simulink model "LimitedSlipDifferentialWithClutches"  (R2023a)
settings: Solver=VariableStepAuto  StartTime=0.0  StopTime=Sim_Time  FixedStep=1e-3  RelTol=1e-3  AbsTol=1e-3  EnableMultiTasking=on
model workspace (MATLAB code in the model file):
  | MFormulaCoeff.DryTarmac = [10 1.9 1 0.97];
  | MFormulaCoeff.WetTarmac = [12 2.3 0.82 1];
  | MFormulaCoeff.Snow         = [5 2 0.3 1];
  | MFormulaCoeff.Ice            = [4 2 0.1 1];
libraries: fl_lib x46, nesl_utility x14, sdl_lib x11, simulink x1
(part 1 of 2)
CloseFcn:
  | try,close(h1_LimitedSlipDifferentialWithClutches),end
  | clear h1_LimitedSlipDifferentialWithClutches
  | try,close(h2_LimitedSlipDifferentialWithClutches),end
  | clear h2_LimitedSlipDifferentialWithClutches
  | 
  | clear simlog_LimitedSlipDifferentialWithClutches
  | clear logsout_LimitedSlipDifferentialWithClutches
Description:
  | Limited Slip Differential with Clutches
settings Model: Creator=The MathWorks, Inc.  LastModifiedBy=MCO
settings SolverCC: AutoScaleAbsTol=off  ZcThreshold=0  MaxConsecutiveZCs=100  MaxConsecutiveMinStep=10  ZeroCrossAlgorithm=Adaptive  AlgebraicLoopSolver=TrustRegion
settings DataIOCC: LimitDataPoints=on  MaxDataPoints=10000  SaveOutput=off  DSMLogging=off  ReturnWorkspaceOutputs=off  SignalLoggingName=logsout_LimitedSlipDifferentialWithClutches
settings OptimizationCC: ExpressionDepthLimit=2147483647  InitFltsAndDblsToZero=on  EfficientMapNaN2IntZero=off  LifeSpan=inf
settings DebuggingCC: SaveWithDisabledLinksMsg=none  SaveWithParameterizedLinksMsg=none  SignalResolutionControl=TryResolveAllWithWarning  MaxConsecutiveZCsMsg=none  IgnoredZcDiagnostic=none  UnconnectedInputMsg=warning  UnconnectedOutputMsg=warning  UnconnectedLineMsg=warning  StateNameClashWarn=warning  SFUnexpectedBacktrackingDiag=warning  SFNoUnconditionalDefaultTransitionDiag=warning  SFExecutionAtInitializationDiag=none  ArithmeticOperatorsInVariantConditions=warning
settings HardwareCC: ProdBitPerPointer=32  ProdBitPerSizeT=32  ProdBitPerPtrDiffT=32  ProdLargestAtomicFloat=None  ProdIntDivRoundTo=Undefined  ProdEndianess=Unspecified  ProdWordSize=32  ProdHWDeviceType=32-bit Generic
settings ModelReferenceCC: EnableRefExpFcnMdlSchedulingChecks=on  PropagateSignalLabelsOutOfModel=off
settings SFSimCC: SimUseLocalCustomCode=off  CustomCodeUndefinedFunction=UseInterfaceOnly
settings RTWCC: RTWUseLocalCustomCode=off  DLArmComputeVersion=19.05
settings CodeAppCC: StateflowObjectComments=on
settings GRTTargetCC: TargetFcnLib=ansi_tfl_tmw.mat  TargetLangStandard=C89/C90 (ANSI)  CombineOutputUpdateFcns=off  GRTInterface=on
settings ConfigComp: CovMetricSettings=dw  CovSaveCumulativeToWorkspaceVar=on  CovSaveSingleToWorkspaceVar=on  CovExternalEMLEnable=off
settings SimscapeCC: SimscapeLogType=all  SimscapeLogSimulationStatistics=on  SimscapeLogName=simlog_LimitedSlipDifferentialWithClutches  SimscapeLogDataHistory=10000

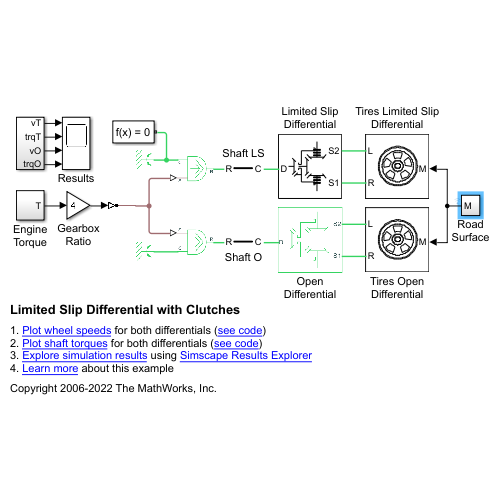
[thumbnail: Simulink's stored preview of the top-level diagram]
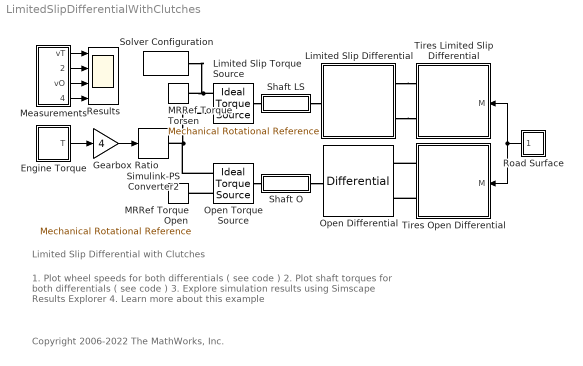
== system LimitedSlipDifferentialWithClutches ==
  note: Limited Slip Differential with Clutches
  note: 1. Plot wheel speeds for both differentials ( see code )
      | 2. Plot shaft torques for both differentials ( see code )
      | 3. Explore simulation results using Simscape Results Explorer
      | 4. Learn more about this example
  note: Copyright 2006-2022 The MathWorks, Inc.
  Engine Torque : Subsystem
  Gearbox Ratio : Gain  Gain=4  SaturateOnIntegerOverflow=on  OutDataTypeStr=Inherit: Same as input  ParamDataTypeStr=Inherit: Same as input
  Limited Slip Differential : Subsystem  Tag=PublishSubsystem
      mask Display:
      | plot([73.6983027309179;73.6983027309179], [209.756707772613;130.389304831624])
      | plot([73.6983027309179;39.6837014704943], [170.073006302118;170.073006302118])
      | plot([62.3601023107767;85.0365031510592], [221.094908192754;198.418507352471])
      | plot([85.0365031510592;62.3601023107767], [141.727505251765;119.051104411483])
      | plot([102.043803781271;119.051104411483;119.051104411483;198.418507352471;198.418507352471], [181.41120672226;181.41120672226;260.778609663248;260.778609663248;277.78591029346])
      | patch([80 120 120 80 80]+115,[150 150 155 155 150]+80,[0 0 0]);
      | patch([80 120 120 80 80]+115,[150 150 155 155 150]+95,[0 0 0]);
      | patch([80 120 120 80 80]+115,[150 150 155 155 150]+110,[0 0 0]);
      | patch([80 120 120 80 80]+115,[150 150 155 155 150]-80,[0 0 0]);
      | patch([80 120 120 80 80]+115,[150 150 155 155 150]-65,[0 0 0]);
      | patch([80 120 120 80 80]+115,[150 150 155 155 150]-50,[0 0 0]);
      | 
      | plot([164.403906092048;255.109509453177], [226.764008402824;226.764008402824])
      | plot([153.065705671906;153.065705671906], [215.425807982683;124.720204621553])
      | plot([209.756707772613;209.756707772613], [317.469611763954;226.764008402824])
      | plot([187.08030693233;198.418507352471], [277.78591029346;277.78591029346])
      | plot([141.727505251765;164.403906092048], [226.764008402824;204.087607562542])
      | plot([175.742106512189;153.065705671906], [124.720204621553;102.043803781271])
      | plot([153.065705671906;175.742106512189], [238.102208822966;215.425807982683])
      | plot([209.756707772613;209.756707772613], [113.382004201412;22.6764008402824])
      | plot([164.403906092048;141.727505251765], [136.058405041695;113.382004201412])
      | plot([243.771309033036;266.447709873319], [124.720204621553;102.043803781271])
      | plot([266.447709873319;243.771309033036], [238.102208822966;215.425807982683])
      | plot([164.403906092048;255.109509453177], [113.382004201412;113.382004201412])
      | plot([187.08030693233;198.418507352471;198.418507352471;119.051104411483;119.051104411483;102.043803781271;102.043803781271], [62.3601023107767;62.3601023107767;79.3674029409885;79.3674029409885;158.734805881977;158.734805881977;147.396605461836])
      | plot([102.043803781271;153.065705671906], [170.073006302118;170.073006302118])
      | plot([102.043803781271;102.043803781271], [181.41120672226;192.749407142401])
      | plot([96.3747035712004;73.6983027309179], [130.389304831624;107.712903991342])
      | plot([85.0365031510592;119.051104411483], [119.051104411483;119.051104411483])
      | plot([-20;-20;360.146012604237;360.146012604237;-20], [360.146012604237;-20;-20;360.146012604237;360.146012604237])
  Limited Slip Torque Source : fl_lib/Mechanical/Mechanical Sources/Ideal Torque Source
  MRRef Torque Open : fl_lib/Mechanical/Rotational Elements/Mechanical Rotational Reference
  MRRef Torque Torsen : fl_lib/Mechanical/Rotational Elements/Mechanical Rotational Reference
  Measurements : Subsystem
  Open Differential : sdl_lib/Gears/Differential  driveshaft_location=2  cd_ratio=1.33  friction_model=1  efficiency=[ 0.9 0.92 ]  temperature_TLU=[ 280 300 320 ] K  efficiency_ss_TLU=[ 0.95 0.9 0.85 ]  efficiency_cd_TLU=[ 0.95 0.9 0.85 ]  pwr_thr=[ 0.001 0.001 ] W  mu_visc=[ 0 0 ] N*m/(rad/s)  model_inertia=0  carrier_inertia=0.001 kg*m^2  planet_inertia=0.001 kg*m^2  thermal_mass=50 J/K  T_init=300 K
  Open Torque Source : fl_lib/Mechanical/Mechanical Sources/Ideal Torque Source
  Results : Scope  NumInputPorts=4
  Road Surface : Subsystem
  Shaft LS : Subsystem
      mask Display:
      | patch([-1 -1 1 1 -1]*25,[-1 1 1 -1 -1]*5,[1 1 1]);
      | patch([-1 -1 1 1 -1]*11,[-1 1 1 -1 -1]*0.1,[0 0 0]);
  Shaft O : Subsystem
      mask Display:
      | patch([-1 -1 1 1 -1]*25,[-1 1 1 -1 -1]*5,[1 1 1]);
      | patch([-1 -1 1 1 -1]*11,[-1 1 1 -1 -1]*0.1,[0 0 0]);
  Simulink-PS Converter2 : nesl_utility/Simulink-PS Converter  PhysicalDomain=network_engine_domain  SubClassName=ps_input  LeftPortType=input  RightPortType=output  PseudoPeriodic=off  Frequencies=[]  NoiseDistribution=none  NoiseParameters=[]  Unit=1  AffineConversion=off  FilteringAndDerivatives=filter  SimscapeFilterOrder=1  InputFilterTimeConstant=0.001  UdotUserProvided=0
  Solver Configuration : nesl_utility/Solver Configuration  PhysicalDomain=network_engine_domain  SubClassName=solver  LeftPortType=input  RightPortType=generic  Tones=[]  Harmonics=[]  SimulateNoise=off  Profile=off  UseLocalSampling=off  EnableSwitchedLinearOptims=on  FrequencyDomain=off  UseCCode=off  RelTol=0.001  AbsTol=1e-06  MinStep=1e-09  ToWorkspace=off  RevertToSquareIcSolve=off  NumHomotopyIterations=100  PhasorMode=off  PhasorModeNumHarmonics=1  ConsistencySolver=NEWTON_XTOL_AFTER_FTOL  IndexReductionMethod=DerivativeReplacement  DoDC=off  ResidualTolerance=1e-9  ConsistencyTolSource=GLOBAL  ConsistencyAbsTol=0.001  ConsistencyRelTol=0.001  ConsistencyTolFactor=0.001  UseLocalSolver=off  LocalSolverChoice=NE_BACKWARD_EULER_ADVANCER  ResolveIndetEquations=on  FunctionEvalNumThread=1  LocalSolverSampleTime=.001  DoFixedCost=off  MaxNonlinIter=12  MaxModeIter=2  ComputeImpulses=off  ImpulseIterations=2  LinearAlgebra=auto  LinearAlgebraNumThread=0  EquationFormulation=NE_TIME_EF  DelaysMemoryBudget=1024  AutomaticFiltering=on  FilteringTimeConstant=0.001  PartitionStorageMethod=AS_NEEDED  PartitionMemoryBudget=1024  PartitionMethod=FAST
  Tires Limited Slip Differential : Subsystem  Tag=PublishSubsystem
      mask Display:
      | plot([199.740630080105;207.645625381422;215.666495494822;223.725995056458;231.746506679781;239.614636200368], [285.533592122614;287.104128914395;287.892278108498;287.890449397339;287.098660392404;285.533592122614])
      | plot([182.29422131887;191.284049604609;200.547323621308;209.994832976365;219.535592990157;229.077720928241;238.529320882316;247.799368778054;256.798588986696;257.061044961602], [327.86290499758;331.09432156677;333.429020721321;334.844518032099;335.327181486212;334.872362770745;333.484442038558;331.176785725016;327.971617821912;327.86290499758])
      | plot([182.293066754937;199.741297401488], [327.862962149084;285.533680580556])
      | plot([239.613968878984;257.062199525535], [285.533680580556;327.862962149084])
      | plot([161.12998329239;162.078783791624;163.80431860203;166.28996988011;169.511799445263;173.438779317544;173.475674844307], [230.482414304504;238.453500201144;246.293204428793;253.926026350122;261.278457717503;268.279690597622;268.338450605791])
      | plot([115.521208412501;115.19363189143;115.795069625231;117.319729439748;119.752928027503;123.071232355974;127.242685340509;132.227113608518;137.976514391014;138.639091794056], [226.950718692202;236.412705455625;245.861238280392;255.205322630308;264.354969865087;273.222063880151;281.72120971289;289.770555942828;297.29258296555;298.068153121848])
      | plot([115.523664280772;161.128425970674], [226.952978409827;230.480418540537])
      | plot([173.474466428161;138.640995137393], [268.337409943342;298.068691045046])
      | plot([197.791294323752;190.505905487348;183.583957764389;177.092113295368;171.092892091325;165.644069931963;165.540704869119], [173.730032993176;177.080059057945;181.128046811489;185.835011918887;191.155623733067;197.038641853715;197.162104079289])
      | plot([187.018154556423;177.935574592276;169.151745387891;160.751260020237;152.815019755577;145.419454926048;138.635788863788;132.529351981303;127.158952603892;126.547993304079], [129.256249226993;131.857994736568;135.337460645285;139.661137794374;144.787386809327;150.666839109836;157.242872356214;164.45215575347;172.225259961496;173.223046112601])
      | plot([187.017316929996;197.78860732913], [129.25548478961;173.726426437497])
      | plot([165.537726134062;126.546914689243], [197.158707305789;173.222506418824])
      | plot([269.470357644972;273.38551933114;276.602305486856;279.089736702965;280.82385765709;281.787967816474;281.81616724833], [262.922159053497;255.989463868491;248.706398553292;241.143103008215;233.372415903877;225.469173204983;225.06588742066])
      | plot([304.431346528147;310.265227080294;315.332070863713;319.583081402952;322.977319142679;325.482095717982;327.073288761189;327.735574213461;327.462573903851;327.423015855416], [292.655530476138;285.116593543042;277.042138363134;268.509926353743;259.602127380701;250.404528417616;241.005707370423;231.496180023723;221.967528324303;221.475771485887])
      | plot([304.430681280792;269.471229985356], [292.651550844312;262.920269742608])
      | plot([281.817270442843;327.422032132745], [225.063278339803;221.472848206758])
      | plot([274.506490288884;269.03580586378;263.012187571475;256.493646148968;249.542958713556;242.227064184873;242.193171590222], [197.094155985096;191.184202827407;185.838928552521;181.109811073729;177.042394377551;173.675849910247;173.662235378073])
      | plot([313.374602600377;308.147922202874;302.181086731703;295.531560074253;288.263380807238;280.446545470191;272.156334460522;263.472587042146;254.478932449722;252.966160341391], [173.157457637183;165.349405231175;158.09125499764;151.452906891035;145.498291832517;140.284756020223;135.862508654033;132.274138393531;129.554203205929;129.189658564058])
      | plot([313.375261612236;274.510430172086], [173.15951641649;197.095717303455])
      | plot([242.196558974683;252.967849373817], [173.663436435163;129.192494787276])
      | plot([371.389053761959;370.658673461755;368.474566522701;364.857767088574;359.843106915069;353.478879920948;345.826377091206;336.959296211375;326.963032117569;315.933854297525;303.977979762811;291.210550120943;277.754522698759;263.739486396147;249.3004136741;234.576360696131;219.709128141403;204.841895586676;190.117842608706;175.678769886659;161.663733584047;148.207706161863;135.440276519995;123.484401985281;112.455224165237;102.458960071431;93.5918791916006;85.939376361858;79.5751493677372;74.5604891942319;70.9436897601051;68.7595828210511;68.0292025208473;68.7595828210511;70.9436897601053;74.5604891942321;79.5751493677375;85.9393763618583;93.5918791916009;102.458960071431;112.455224165237;123.484401985282;135.440276519995;148.207706161863;161.663733584048;175.67876988666;190.117842608707;204.841895586676;219.709128141403;234.576360696131;249.3004136741;263.739486396147;277.754522698759;291.210550120943;303.977979762811;315.933854297525;326.963032117569;336.959296211375;345.826377091205;353.478879920948;359.843106915069;364.857767088574;368.474566522701;370.658673461755;371.389053761959;371.389053761959;371.389053761959], [228.149788454175;213.282555899448;198.558502921478;184.119430199431;170.104393896819;156.648366474635;143.880936832767;131.925062298053;120.895884478009;110.899620384203;102.032539504372;94.3800366746299;88.0158096805091;83.0011495070038;79.3843500728769;77.2002431338229;76.4698628336191;77.2002431338229;79.3843500728769;83.0011495070038;88.0158096805092;94.38003667463;102.032539504373;110.899620384203;120.895884478009;131.925062298053;143.880936832767;156.648366474635;170.104393896819;184.119430199431;198.558502921479;213.282555899448;228.149788454175;243.017021008903;257.741073986872;272.180146708919;286.195183011531;299.651210433715;312.418640075584;324.374514610297;335.403692430341;345.399956524147;354.267037403978;361.91954023372;368.283767227841;373.298427401346;376.915226835473;379.099333774527;379.829714074731;379.099333774527;376.915226835473;373.298427401346;368.283767227841;361.91954023372;354.267037403978;345.399956524147;335.403692430341;324.374514610297;312.418640075583;299.651210433715;286.195183011531;272.180146708919;257.741073986872;243.017021008903;228.149788454176;228.149788454175;228.149788454175])
      | plot([363.45231346786;362.760150741504;360.690328467866;357.26278016692;352.510515002494;346.479299885972;339.227218715925;330.824112998412;321.350909235096;310.898839556798;299.568563108203;287.46919664527;274.717263681223;261.435572301422;247.752032454366;233.798424108965;219.709128141403;205.619832173842;191.666223828441;177.982683981384;164.700992601583;151.949059637537;139.849693174603;128.519416726008;118.067347047711;108.594143284395;100.191037566881;92.9389563968342;86.9077412803127;82.1554761158862;78.7279278149405;76.6581055413021;75.9659428149462;76.6581055413021;78.7279278149406;82.1554761158864;86.907741280313;92.9389563968345;100.191037566881;108.594143284395;118.067347047711;128.519416726009;139.849693174604;151.949059637537;164.700992601584;177.982683981384;191.666223828441;205.619832173842;219.709128141403;233.798424108965;247.752032454366;261.435572301422;274.717263681223;287.46919664527;299.568563108203;310.898839556798;321.350909235095;330.824112998411;339.227218715925;346.479299885972;352.510515002493;357.26278016692;360.690328467866;362.760150741504;363.45231346786;363.45231346786;363.45231346786], [228.149788454175;214.060492486614;200.106884141213;186.423344294156;173.141652914355;160.389719950309;148.290353487375;136.96007703878;126.508007360483;117.034803597167;108.631697879653;101.379616709606;95.3484015930846;90.596136428658;87.1685881277123;85.0987658540739;84.406603127718;85.0987658540739;87.1685881277124;90.5961364286582;95.3484015930846;101.379616709606;108.631697879653;117.034803597167;126.508007360483;136.960077038781;148.290353487376;160.389719950309;173.141652914355;186.423344294156;200.106884141213;214.060492486614;228.149788454175;242.239084421737;256.192692767138;269.876232614194;283.157923993995;295.909856958042;308.009223420975;319.33949986957;329.791569547868;339.264773311184;347.667879028697;354.919960198744;360.951175315265;365.703440479692;369.130988780638;371.200811054276;371.892973780632;371.200811054276;369.130988780638;365.703440479692;360.951175315265;354.919960198744;347.667879028697;339.264773311184;329.791569547868;319.33949986957;308.009223420975;295.909856958042;283.157923993995;269.876232614194;256.192692767138;242.239084421737;228.149788454176;228.149788454175;228.149788454175])
      | plot([261.408509686589;261.209838965396;260.615740109466;259.631934615548;258.267897068353;256.536763895118;254.455206854636;252.043272479101;249.324189015046;246.324142722634;243.072025687652;239.599157574934;235.93898400287;232.126754443812;228.199182752392;224.194093591025;220.150058157742;216.106022724459;212.100933563092;208.173361871672;204.361132312614;200.70095874055;197.228090627832;193.97597359285;190.975927300438;188.256843836383;185.844909460848;183.763352420366;182.032219247131;180.668181699936;179.684376206018;179.090277350088;178.891606628895;179.090277350088;179.684376206019;180.668181699936;182.032219247131;183.763352420366;185.844909460848;188.256843836383;190.975927300438;193.97597359285;197.228090627833;200.70095874055;204.361132312614;208.173361871672;212.100933563092;216.106022724459;220.150058157742;224.194093591025;228.199182752392;232.126754443812;235.93898400287;239.599157574934;243.072025687652;246.324142722634;249.324189015046;252.043272479101;254.455206854636;256.536763895118;258.267897068353;259.631934615548;260.615740109465;261.209838965396;261.408509686589;261.408509686589], [229.220618493855;225.176583060572;221.171493899205;217.243922207785;213.431692648727;209.771519076663;206.298650963945;203.046533928963;200.046487636551;197.327404172496;194.915469796961;192.833912756479;191.102779583244;189.738742036049;188.754936542131;188.160837686201;187.962166965008;188.160837686201;188.754936542131;189.738742036049;191.102779583244;192.833912756479;194.915469796961;197.327404172496;200.046487636551;203.046533928963;206.298650963945;209.771519076663;213.431692648727;217.243922207785;221.171493899205;225.176583060572;229.220618493855;233.264653927138;237.269743088505;241.197314779925;245.009544338983;248.669717911047;252.142586023765;255.394703058747;258.394749351159;261.113832815214;263.525767190749;265.607324231231;267.338457404466;268.702494951661;269.686300445579;270.280399301509;270.479070022702;270.280399301509;269.686300445579;268.702494951661;267.338457404466;265.607324231231;263.525767190749;261.113832815214;258.394749351159;255.394703058747;252.142586023765;248.669717911047;245.009544338983;241.197314779925;237.269743088505;233.264653927139;229.220618493855;229.220618493855])
      | plot([240.243868902326;240.144988512846;239.849299616612;239.359649859334;238.680754835845;237.819152676342;236.783141080621;235.58269740669;234.229382583359;232.736229772174;231.117618850946;229.38913792767;227.56743321852;225.670048735692;223.715257328969;221.721884708198;219.709128141403;217.696371574609;215.702998953837;213.748207547115;211.850823064286;210.029118355137;208.30063743186;206.682026510633;205.188873699447;203.835558876116;202.635115202186;201.599103606465;200.737501446962;200.058606423472;199.568956666194;199.27326776996;199.174387380481;199.27326776996;199.568956666194;200.058606423472;200.737501446962;201.599103606465;202.635115202186;203.835558876116;205.188873699447;206.682026510633;208.30063743186;210.029118355137;211.850823064286;213.748207547115;215.702998953837;217.696371574609;219.709128141403;221.721884708198;223.715257328969;225.670048735692;227.56743321852;229.38913792767;231.117618850946;232.736229772174;234.229382583359;235.58269740669;236.783141080621;237.819152676342;238.680754835845;239.359649859334;239.849299616612;240.144988512846;240.243868902326;240.243868902326], [230.66938854754;228.656631980745;226.663259359974;224.708467953251;222.811083470423;220.989378761273;219.260897837997;217.642286916769;216.149134105584;214.795819282253;213.595375608322;212.559364012601;211.697761853098;211.018866829609;210.529217072331;210.233528176097;210.134647786617;210.233528176097;210.529217072331;211.018866829609;211.697761853098;212.559364012601;213.595375608322;214.795819282253;216.149134105584;217.642286916769;219.260897837997;220.989378761273;222.811083470423;224.708467953251;226.663259359974;228.656631980745;230.66938854754;232.682145114334;234.675517735106;236.630309141828;238.527693624657;240.349398333806;242.077879257083;243.69649017831;245.189642989496;246.542957812827;247.743401486757;248.779413082478;249.641015241981;250.319910265471;250.809560022749;251.105248918983;251.204129308462;251.105248918983;250.809560022749;250.319910265471;249.641015241981;248.779413082478;247.743401486757;246.542957812827;245.189642989496;243.69649017831;242.077879257083;240.349398333806;238.527693624657;236.630309141828;234.675517735106;232.682145114334;230.66938854754;230.66938854754])
      | plot([339.327142573893;338.751149139472;337.02871596785;334.17643103205;330.22176339522;325.202798668544;319.167872225986;312.175103708213;304.291837298687;295.593993162365;286.165336293004;276.096669810484;265.484960477125;254.432404854758;243.045445095968;231.433743847976;219.709128141403;207.98451243483;196.372811186839;184.985851428048;173.933295805681;163.321586472322;153.252919989803;143.824263120442;135.126418984119;127.243152574594;120.250384056821;114.215457614262;109.196492887586;105.241825250756;102.389540314956;100.667107143335;100.091113708913;100.667107143335;102.389540314956;105.241825250756;109.196492887586;114.215457614262;120.250384056821;127.243152574594;135.12641898412;143.824263120442;153.252919989803;163.321586472323;173.933295805681;184.985851428048;196.372811186839;207.984512434831;219.709128141403;231.433743847976;243.045445095968;254.432404854758;265.484960477125;276.096669810484;286.165336293004;295.593993162365;304.291837298687;312.175103708212;319.167872225986;325.202798668544;330.22176339522;334.17643103205;337.02871596785;338.751149139472;339.327142573893;339.327142573893;339.327142573893], [228.149788454175;216.425172747602;204.813471499611;193.42651174082;182.373956118453;171.762246785094;161.693580302574;152.264923433213;143.567079296891;135.683812887366;128.691044369592;122.656117927034;117.637153200358;113.682485563528;110.830200627728;109.107767456107;108.531774021685;109.107767456107;110.830200627728;113.682485563528;117.637153200358;122.656117927034;128.691044369592;135.683812887366;143.567079296891;152.264923433214;161.693580302575;171.762246785094;182.373956118453;193.42651174082;204.813471499611;216.425172747602;228.149788454175;239.874404160748;251.48610540874;262.87306516753;273.925620789897;284.537330123256;294.605996605776;304.034653475137;312.732497611459;320.615764020985;327.608532538758;333.643458981316;338.662423707992;342.617091344822;345.469376280622;347.191809452243;347.767802886665;347.191809452243;345.469376280622;342.617091344822;338.662423707992;333.643458981316;327.608532538758;320.615764020985;312.732497611459;304.034653475137;294.605996605776;284.537330123256;273.925620789897;262.87306516753;251.48610540874;239.874404160748;228.149788454176;228.149788454175;228.149788454175])
      | plot([-20;467.858916595578;467.858916595578;-20;-20], [473.528016805649;473.528016805649;-20;-20;473.528016805649])
  Tires Open Differential : Subsystem
      mask Display:
      | plot([199.740630080105;207.645625381422;215.666495494822;223.725995056458;231.746506679781;239.614636200368], [285.533592122614;287.104128914395;287.892278108498;287.890449397339;287.098660392404;285.533592122614])
      | plot([182.29422131887;191.284049604609;200.547323621308;209.994832976365;219.535592990157;229.077720928241;238.529320882316;247.799368778054;256.798588986696;257.061044961602], [327.86290499758;331.09432156677;333.429020721321;334.844518032099;335.327181486212;334.872362770745;333.484442038558;331.176785725016;327.971617821912;327.86290499758])
      | plot([182.293066754937;199.741297401488], [327.862962149084;285.533680580556])
      | plot([239.613968878984;257.062199525535], [285.533680580556;327.862962149084])
      | plot([161.12998329239;162.078783791624;163.80431860203;166.28996988011;169.511799445263;173.438779317544;173.475674844307], [230.482414304504;238.453500201144;246.293204428793;253.926026350122;261.278457717503;268.279690597622;268.338450605791])
      | plot([115.521208412501;115.19363189143;115.795069625231;117.319729439748;119.752928027503;123.071232355974;127.242685340509;132.227113608518;137.976514391014;138.639091794056], [226.950718692202;236.412705455625;245.861238280392;255.205322630308;264.354969865087;273.222063880151;281.72120971289;289.770555942828;297.29258296555;298.068153121848])
      | plot([115.523664280772;161.128425970674], [226.952978409827;230.480418540537])
      | plot([173.474466428161;138.640995137393], [268.337409943342;298.068691045046])
      | plot([197.791294323752;190.505905487348;183.583957764389;177.092113295368;171.092892091325;165.644069931963;165.540704869119], [173.730032993176;177.080059057945;181.128046811489;185.835011918887;191.155623733067;197.038641853715;197.162104079289])
      | plot([187.018154556423;177.935574592276;169.151745387891;160.751260020237;152.815019755577;145.419454926048;138.635788863788;132.529351981303;127.158952603892;126.547993304079], [129.256249226993;131.857994736568;135.337460645285;139.661137794374;144.787386809327;150.666839109836;157.242872356214;164.45215575347;172.225259961496;173.223046112601])
      | plot([187.017316929996;197.78860732913], [129.25548478961;173.726426437497])
      | plot([165.537726134062;126.546914689243], [197.158707305789;173.222506418824])
      | plot([269.470357644972;273.38551933114;276.602305486856;279.089736702965;280.82385765709;281.787967816474;281.81616724833], [262.922159053497;255.989463868491;248.706398553292;241.143103008215;233.372415903877;225.469173204983;225.06588742066])
      | plot([304.431346528147;310.265227080294;315.332070863713;319.583081402952;322.977319142679;325.482095717982;327.073288761189;327.735574213461;327.462573903851;327.423015855416], [292.655530476138;285.116593543042;277.042138363134;268.509926353743;259.602127380701;250.404528417616;241.005707370423;231.496180023723;221.967528324303;221.475771485887])
      | plot([304.430681280792;269.471229985356], [292.651550844312;262.920269742608])
      | plot([281.817270442843;327.422032132745], [225.063278339803;221.472848206758])
      | plot([274.506490288884;269.03580586378;263.012187571475;256.493646148968;249.542958713556;242.227064184873;242.193171590222], [197.094155985096;191.184202827407;185.838928552521;181.109811073729;177.042394377551;173.675849910247;173.662235378073])
      | plot([313.374602600377;308.147922202874;302.181086731703;295.531560074253;288.263380807238;280.446545470191;272.156334460522;263.472587042146;254.478932449722;252.966160341391], [173.157457637183;165.349405231175;158.09125499764;151.452906891035;145.498291832517;140.284756020223;135.862508654033;132.274138393531;129.554203205929;129.189658564058])
      | plot([313.375261612236;274.510430172086], [173.15951641649;197.095717303455])
      | plot([242.196558974683;252.967849373817], [173.663436435163;129.192494787276])
      | plot([371.389053761959;370.658673461755;368.474566522701;364.857767088574;359.843106915069;353.478879920948;345.826377091206;336.959296211375;326.963032117569;315.933854297525;303.977979762811;291.210550120943;277.754522698759;263.739486396147;249.3004136741;234.576360696131;219.709128141403;204.841895586676;190.117842608706;175.678769886659;161.663733584047;148.207706161863;135.440276519995;123.484401985281;112.455224165237;102.458960071431;93.5918791916006;85.939376361858;79.5751493677372;74.5604891942319;70.9436897601051;68.7595828210511;68.0292025208473;68.7595828210511;70.9436897601053;74.5604891942321;79.5751493677375;85.9393763618583;93.5918791916009;102.458960071431;112.455224165237;123.484401985282;135.440276519995;148.207706161863;161.663733584048;175.67876988666;190.117842608707;204.841895586676;219.709128141403;234.576360696131;249.3004136741;263.739486396147;277.754522698759;291.210550120943;303.977979762811;315.933854297525;326.963032117569;336.959296211375;345.826377091205;353.478879920948;359.843106915069;364.857767088574;368.474566522701;370.658673461755;371.389053761959;371.389053761959;371.389053761959], [228.149788454175;213.282555899448;198.558502921478;184.119430199431;170.104393896819;156.648366474635;143.880936832767;131.925062298053;120.895884478009;110.899620384203;102.032539504372;94.3800366746299;88.0158096805091;83.0011495070038;79.3843500728769;77.2002431338229;76.4698628336191;77.2002431338229;79.3843500728769;83.0011495070038;88.0158096805092;94.38003667463;102.032539504373;110.899620384203;120.895884478009;131.925062298053;143.880936832767;156.648366474635;170.104393896819;184.119430199431;198.558502921479;213.282555899448;228.149788454175;243.017021008903;257.741073986872;272.180146708919;286.195183011531;299.651210433715;312.418640075584;324.374514610297;335.403692430341;345.399956524147;354.267037403978;361.91954023372;368.283767227841;373.298427401346;376.915226835473;379.099333774527;379.829714074731;379.099333774527;376.915226835473;373.298427401346;368.283767227841;361.91954023372;354.267037403978;345.399956524147;335.403692430341;324.374514610297;312.418640075583;299.651210433715;286.195183011531;272.180146708919;257.741073986872;243.017021008903;228.149788454176;228.149788454175;228.149788454175])
      | plot([363.45231346786;362.760150741504;360.690328467866;357.26278016692;352.510515002494;346.479299885972;339.227218715925;330.824112998412;321.350909235096;310.898839556798;299.568563108203;287.46919664527;274.717263681223;261.435572301422;247.752032454366;233.798424108965;219.709128141403;205.619832173842;191.666223828441;177.982683981384;164.700992601583;151.949059637537;139.849693174603;128.519416726008;118.067347047711;108.594143284395;100.191037566881;92.9389563968342;86.9077412803127;82.1554761158862;78.7279278149405;76.6581055413021;75.9659428149462;76.6581055413021;78.7279278149406;82.1554761158864;86.907741280313;92.9389563968345;100.191037566881;108.594143284395;118.067347047711;128.519416726009;139.849693174604;151.949059637537;164.700992601584;177.982683981384;191.666223828441;205.619832173842;219.709128141403;233.798424108965;247.752032454366;261.435572301422;274.717263681223;287.46919664527;299.568563108203;310.898839556798;321.350909235095;330.824112998411;339.227218715925;346.479299885972;352.510515002493;357.26278016692;360.690328467866;362.760150741504;363.45231346786;363.45231346786;363.45231346786], [228.149788454175;214.060492486614;200.106884141213;186.423344294156;173.141652914355;160.389719950309;148.290353487375;136.96007703878;126.508007360483;117.034803597167;108.631697879653;101.379616709606;95.3484015930846;90.596136428658;87.1685881277123;85.0987658540739;84.406603127718;85.0987658540739;87.1685881277124;90.5961364286582;95.3484015930846;101.379616709606;108.631697879653;117.034803597167;126.508007360483;136.960077038781;148.290353487376;160.389719950309;173.141652914355;186.423344294156;200.106884141213;214.060492486614;228.149788454175;242.239084421737;256.192692767138;269.876232614194;283.157923993995;295.909856958042;308.009223420975;319.33949986957;329.791569547868;339.264773311184;347.667879028697;354.919960198744;360.951175315265;365.703440479692;369.130988780638;371.200811054276;371.892973780632;371.200811054276;369.130988780638;365.703440479692;360.951175315265;354.919960198744;347.667879028697;339.264773311184;329.791569547868;319.33949986957;308.009223420975;295.909856958042;283.157923993995;269.876232614194;256.192692767138;242.239084421737;228.149788454176;228.149788454175;228.149788454175])
      | plot([261.408509686589;261.209838965396;260.615740109466;259.631934615548;258.267897068353;256.536763895118;254.455206854636;252.043272479101;249.324189015046;246.324142722634;243.072025687652;239.599157574934;235.93898400287;232.126754443812;228.199182752392;224.194093591025;220.150058157742;216.106022724459;212.100933563092;208.173361871672;204.361132312614;200.70095874055;197.228090627832;193.97597359285;190.975927300438;188.256843836383;185.844909460848;183.763352420366;182.032219247131;180.668181699936;179.684376206018;179.090277350088;178.891606628895;179.090277350088;179.684376206019;180.668181699936;182.032219247131;183.763352420366;185.844909460848;188.256843836383;190.975927300438;193.97597359285;197.228090627833;200.70095874055;204.361132312614;208.173361871672;212.100933563092;216.106022724459;220.150058157742;224.194093591025;228.199182752392;232.126754443812;235.93898400287;239.599157574934;243.072025687652;246.324142722634;249.324189015046;252.043272479101;254.455206854636;256.536763895118;258.267897068353;259.631934615548;260.615740109465;261.209838965396;261.408509686589;261.408509686589], [229.220618493855;225.176583060572;221.171493899205;217.243922207785;213.431692648727;209.771519076663;206.298650963945;203.046533928963;200.046487636551;197.327404172496;194.915469796961;192.833912756479;191.102779583244;189.738742036049;188.754936542131;188.160837686201;187.962166965008;188.160837686201;188.754936542131;189.738742036049;191.102779583244;192.833912756479;194.915469796961;197.327404172496;200.046487636551;203.046533928963;206.298650963945;209.771519076663;213.431692648727;217.243922207785;221.171493899205;225.176583060572;229.220618493855;233.264653927138;237.269743088505;241.197314779925;245.009544338983;248.669717911047;252.142586023765;255.394703058747;258.394749351159;261.113832815214;263.525767190749;265.607324231231;267.338457404466;268.702494951661;269.686300445579;270.280399301509;270.479070022702;270.280399301509;269.686300445579;268.702494951661;267.338457404466;265.607324231231;263.525767190749;261.113832815214;258.394749351159;255.394703058747;252.142586023765;248.669717911047;245.009544338983;241.197314779925;237.269743088505;233.264653927139;229.220618493855;229.220618493855])
      | plot([240.243868902326;240.144988512846;239.849299616612;239.359649859334;238.680754835845;237.819152676342;236.783141080621;235.58269740669;234.229382583359;232.736229772174;231.117618850946;229.38913792767;227.56743321852;225.670048735692;223.715257328969;221.721884708198;219.709128141403;217.696371574609;215.702998953837;213.748207547115;211.850823064286;210.029118355137;208.30063743186;206.682026510633;205.188873699447;203.835558876116;202.635115202186;201.599103606465;200.737501446962;200.058606423472;199.568956666194;199.27326776996;199.174387380481;199.27326776996;199.568956666194;200.058606423472;200.737501446962;201.599103606465;202.635115202186;203.835558876116;205.188873699447;206.682026510633;208.30063743186;210.029118355137;211.850823064286;213.748207547115;215.702998953837;217.696371574609;219.709128141403;221.721884708198;223.715257328969;225.670048735692;227.56743321852;229.38913792767;231.117618850946;232.736229772174;234.229382583359;235.58269740669;236.783141080621;237.819152676342;238.680754835845;239.359649859334;239.849299616612;240.144988512846;240.243868902326;240.243868902326], [230.66938854754;228.656631980745;226.663259359974;224.708467953251;222.811083470423;220.989378761273;219.260897837997;217.642286916769;216.149134105584;214.795819282253;213.595375608322;212.559364012601;211.697761853098;211.018866829609;210.529217072331;210.233528176097;210.134647786617;210.233528176097;210.529217072331;211.018866829609;211.697761853098;212.559364012601;213.595375608322;214.795819282253;216.149134105584;217.642286916769;219.260897837997;220.989378761273;222.811083470423;224.708467953251;226.663259359974;228.656631980745;230.66938854754;232.682145114334;234.675517735106;236.630309141828;238.527693624657;240.349398333806;242.077879257083;243.69649017831;245.189642989496;246.542957812827;247.743401486757;248.779413082478;249.641015241981;250.319910265471;250.809560022749;251.105248918983;251.204129308462;251.105248918983;250.809560022749;250.319910265471;249.641015241981;248.779413082478;247.743401486757;246.542957812827;245.189642989496;243.69649017831;242.077879257083;240.349398333806;238.527693624657;236.630309141828;234.675517735106;232.682145114334;230.66938854754;230.66938854754])
      | plot([339.327142573893;338.751149139472;337.02871596785;334.17643103205;330.22176339522;325.202798668544;319.167872225986;312.175103708213;304.291837298687;295.593993162365;286.165336293004;276.096669810484;265.484960477125;254.432404854758;243.045445095968;231.433743847976;219.709128141403;207.98451243483;196.372811186839;184.985851428048;173.933295805681;163.321586472322;153.252919989803;143.824263120442;135.126418984119;127.243152574594;120.250384056821;114.215457614262;109.196492887586;105.241825250756;102.389540314956;100.667107143335;100.091113708913;100.667107143335;102.389540314956;105.241825250756;109.196492887586;114.215457614262;120.250384056821;127.243152574594;135.12641898412;143.824263120442;153.252919989803;163.321586472323;173.933295805681;184.985851428048;196.372811186839;207.984512434831;219.709128141403;231.433743847976;243.045445095968;254.432404854758;265.484960477125;276.096669810484;286.165336293004;295.593993162365;304.291837298687;312.175103708212;319.167872225986;325.202798668544;330.22176339522;334.17643103205;337.02871596785;338.751149139472;339.327142573893;339.327142573893;339.327142573893], [228.149788454175;216.425172747602;204.813471499611;193.42651174082;182.373956118453;171.762246785094;161.693580302574;152.264923433213;143.567079296891;135.683812887366;128.691044369592;122.656117927034;117.637153200358;113.682485563528;110.830200627728;109.107767456107;108.531774021685;109.107767456107;110.830200627728;113.682485563528;117.637153200358;122.656117927034;128.691044369592;135.683812887366;143.567079296891;152.264923433214;161.693580302575;171.762246785094;182.373956118453;193.42651174082;204.813471499611;216.425172747602;228.149788454175;239.874404160748;251.48610540874;262.87306516753;273.925620789897;284.537330123256;294.605996605776;304.034653475137;312.732497611459;320.615764020985;327.608532538758;333.643458981316;338.662423707992;342.617091344822;345.469376280622;347.191809452243;347.767802886665;347.191809452243;345.469376280622;342.617091344822;338.662423707992;333.643458981316;327.608532538758;320.615764020985;312.732497611459;304.034653475137;294.605996605776;284.537330123256;273.925620789897;262.87306516753;251.48610540874;239.874404160748;228.149788454176;228.149788454175;228.149788454175])
      | plot([-20;467.858916595578;467.858916595578;-20;-20], [473.528016805649;473.528016805649;-20;-20;473.528016805649])
  wires:
  Gearbox Ratio/1 -> Simulink-PS Converter2/1
  Road Surface/1(M) -> Tires Open Differential/1(M), Tires Limited Slip Differential/1(M)
  Measurements/1(vT) -> Results/1
  Measurements/2(trqT) -> Results/2
  Measurements/3(vO) -> Results/3
  Measurements/4(trqO) -> Results/4
  Engine Torque/1(T) -> Gearbox Ratio/1
  connections:
  Simulink-PS Converter2/RConn1 -- Limited Slip Torque Source/RConn1 -- Open Torque Source/RConn1
  MRRef Torque Torsen/LConn1 -- Limited Slip Torque Source/RConn2 -- Solver Configuration/RConn1
  Tires Open Differential/RConn2 -- Open Differential/RConn1
  Open Torque Source/RConn2 -- MRRef Torque Open/LConn1
  Tires Open Differential/RConn1 -- Open Differential/RConn2
  Limited Slip Differential/RConn2 -- Tires Limited Slip Differential/RConn2
  Limited Slip Differential/RConn1 -- Tires Limited Slip Differential/RConn1
  Limited Slip Torque Source/LConn1 -- Shaft LS/LConn1
  Shaft LS/RConn1 -- Limited Slip Differential/LConn1
  Open Torque Source/LConn1 -- Shaft O/LConn1
  Shaft O/RConn1 -- Open Differential/LConn1

== system LimitedSlipDifferentialWithClutches/Engine Torque ==
  Repeating Sequence : simulink/Sources/Repeating Sequence  rep_seq_t=[0 0.5 2 6.05 8.4 9.35 12.65 13.25 16 20 30]  rep_seq_y=[0 0 58 185 185 300 300 185 185 99 0]
  T : Outport
  wires:
  Repeating Sequence/1 -> T/1

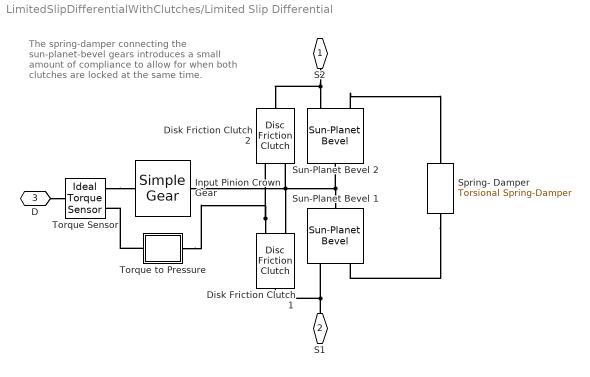
== system LimitedSlipDifferentialWithClutches/Limited Slip Differential ==
  note: The spring-damper connecting the
      | sun-planet-bevel gears introduces a
      | small amount of compliance to allow
      | for when both clutches are locked
      | at the same time.
  Disk Friction Clutch 1 : sdl_lib/Clutches/Disc Friction Clutch  geometry_model=2  r_eff=130 mm  d_o=300 mm  d_i=100 mm  nS=FrictionFaces  piston_area=0.04 m^2  unidirectional=0  friction_model=1  mu_w_vector=[ 0 0.1 0.2 0.3 0.4 0.5 1 2 5 10 100 1000 ] rad/s  temperature_TLU=[280.0, 300.0, 320.0] K  mu_static=0.25  mu_static_vector=[0.4, 0.38, 0.36]  mu_coulomb=0.2  mu_coulomb_vector=[ 0.29 0.28 0.26 0.22 0.21 0.2 0.2 0.19 0.19 0.19 0.19 0.19 ]  mu_coulomb_temp_vector=[0.3, 0.28, 0.25]  mu_coulomb_matrix=[0.34, 0.32, 0.3; 0.3, 0.28, 0.25; 0.25, 0.2, 0.15]  mu_interp_method=1  mu_extrap_method=1  d_f=1  w_tol=0.01 rad/s  pressure_min=100 Pa  mu_visc=0.0032 N*m/(rad/s)  initial_state_locked=0  enable_faults=simscape.enum.onoff.off  fault_type=sdl.enum.clutchFault.lock  external_fault=simscape.enum.onoff.off  temporal_fault=simscape.enum.onoff.off  fault_time=5 s  report_fault=simscape.enum.assert.action.none  thermal_mass=25 kJ/K  T_init=300 K
      settings: InternalSimscapePortConfiguration="{\"Bottom\":[],\"Left\":[{\"id\":\"P\",\"label\":\"P\",\"type\":\"input\"},{\"id\":\"B\",\"label\":\"B\",\"type\":\"foundation.mechanical.rotational.rotational\"}],\"Right\":[{\"id\":\"F\",\"label\":\"F\",\"type\":\"foundation.mechanical.rotational.rotational\"}],\"Top\":[]}"
  Disk Friction Clutch 2 : sdl_lib/Clutches/Disc Friction Clutch  geometry_model=2  r_eff=130 mm  d_o=300 mm  d_i=100 mm  nS=FrictionFaces  piston_area=0.04 m^2  unidirectional=0  friction_model=1  mu_w_vector=[ 0 0.1 0.2 0.3 0.4 0.5 1 2 5 10 100 1000 ] rad/s  temperature_TLU=[280.0, 300.0, 320.0] K  mu_static=0.25  mu_static_vector=[0.4, 0.38, 0.36]  mu_coulomb=0.2  mu_coulomb_vector=[ 0.29 0.28 0.26 0.22 0.21 0.2 0.2 0.19 0.19 0.19 0.19 0.19 ]  mu_coulomb_temp_vector=[0.3, 0.28, 0.25]  mu_coulomb_matrix=[0.34, 0.32, 0.3; 0.3, 0.28, 0.25; 0.25, 0.2, 0.15]  mu_interp_method=1  mu_extrap_method=1  d_f=1  w_tol=0.01 rad/s  pressure_min=100 Pa  mu_visc=0.0032 N*m/(rad/s)  initial_state_locked=0  enable_faults=simscape.enum.onoff.off  fault_type=sdl.enum.clutchFault.lock  external_fault=simscape.enum.onoff.off  temporal_fault=simscape.enum.onoff.off  fault_time=5 s  report_fault=simscape.enum.assert.action.none  thermal_mass=25 kJ/K  T_init=300 K
      settings: InternalSimscapePortConfiguration="{\"Bottom\":[],\"Left\":[{\"id\":\"P\",\"label\":\"P\",\"type\":\"input\"},{\"id\":\"B\",\"label\":\"B\",\"type\":\"foundation.mechanical.rotational.rotational\"}],\"Right\":[{\"id\":\"F\",\"label\":\"F\",\"type\":\"foundation.mechanical.rotational.rotational\"}],\"Top\":[]}"
  Input Pinion Crown Gear : sdl_lib/Gears/Simple Gear  ratio=1.33  rotation_direction=3-2*(1)  friction_model=2  T_noload=0.1 N*m  T_nom=5 N*m  efficiency_nom=0.8  efficiency=0.85  temperature_TLU=[ 280 300 320 ] K  load_TLU=[ 1 5 10 ] N*m  efficiency_TLU=[ 0.95 0.9 0.85 ]  efficiency_TLU2=[ 0.85 0.8 0.75; 0.95 0.9 0.85; 0.85 0.8 0.7 ]  w_thr=0.01 rad/s  pwr_thr=0.001 W  enable_backlash=false  hardstop_model=simscape.enum.hardstop.smooth  backlash_distance=1e-3 mm  r_base=0.1 m  transition=1e-4 mm  backlash_stiffness=1e7 N/m  backlash_damping=1e6 N*s/m  coeff_rest=0  v_tol=0.001 m/s  f_tol=0 N  mu_visc=[ 0 0 ] N*m/(rad/s)  enable_faults=simscape.enum.onoff.off  efficiency_fault=0.05  external_fault=simscape.enum.onoff.off  temporal_fault=simscape.enum.onoff.off  fault_time=5 s  fault_angles=pi / 12 rad  report_fault=simscape.enum.assert.action.none  thermal_mass=50 J/K  temperature_specify=off  temperature_priority=High  temperature=300 K  temperature_nominal_specify=off  temperature_nominal_unit=K  temperature_nominal_value=1  x_backlash_specify=off  x_backlash_priority=None  x_backlash=0 mm  x_backlash_nominal_specify=off  x_backlash_nominal_unit=mm  x_backlash_nominal_value=1  f_hardstop_specify=off  f_hardstop_priority=None  f_hardstop=0 N  f_hardstop_nominal_specify=off  f_hardstop_nominal_unit=N  f_hardstop_nominal_value=1  v_backlash_specify=off  v_backlash_priority=None  v_backlash=0 m/s  v_backlash_nominal_specify=off  v_backlash_nominal_unit=m/s  v_backlash_nominal_value=1
  Spring- Damper : sdl_lib/Couplings & Drives/Torsional Spring-Damper  k=50000 N*m/rad  mu_visc=10000 N*m/(rad/s)  trq_coulomb=0 N*m  static_kinetic_ratio=1.1  w_tol=0.001 rad/s  model_hardstop=0  upper_bound=10 deg  lower_bound=-10 deg  hardstop_model=3  k_endstop=1e+6 N*m/rad  D_endstop=10 N*m/(rad/s)  transition=0.001 rad  coeff_rest=0.7  w_tol_hardstop=0.1 rad/s  trq_tol=0.001 N*m  x0=0 deg
      settings: InternalSimscapePortConfiguration="{\"Bottom\":[],\"Left\":[{\"id\":\"R\",\"label\":\"R\",\"type\":\"foundation.mechanical.rotational.rotational\"}],\"Right\":[{\"id\":\"C\",\"label\":\"C\",\"type\":\"foundation.mechanical.rotational.rotational\"}],\"Top\":[]}"
  Sun-Planet Bevel 1 : sdl_lib/Gears/Planetary Subcomponents/Sun-Planet Bevel  ratio=2  assembly_orientation=1  friction_model=1  efficiency=0.92  temperature_TLU=[ 280 300 320 ] K  efficiency_TLU=[ 0.95 0.9 0.85 ]  pwr_thr=0.001 W  mu_visc=0 N*m/(rad/s)  thermal_mass=50 J/K  temperature_specify=off  temperature_priority=High  temperature=300 K  temperature_nominal_specify=off  temperature_nominal_unit=K  temperature_nominal_value=1
      settings: InternalSimscapePortConfiguration="{\"Bottom\":[],\"Left\":[{\"id\":\"C\",\"label\":\"C\",\"type\":\"foundation.mechanical.rotational.rotational\"}],\"Right\":[{\"id\":\"P\",\"label\":\"P\",\"type\":\"foundation.mechanical.rotational.rotational\"},{\"id\":\"S\",\"label\":\"S\",\"type\":\"foundation.mechanical.rotational.rotational\"}],\"Top\":[]}"
  Sun-Planet Bevel 2 : sdl_lib/Gears/Planetary Subcomponents/Sun-Planet Bevel  ratio=2  assembly_orientation=2  friction_model=1  efficiency=0.92  temperature_TLU=[ 280 300 320 ] K  efficiency_TLU=[ 0.95 0.9 0.85 ]  pwr_thr=0.001 W  mu_visc=0 N*m/(rad/s)  thermal_mass=50 J/K  temperature_specify=off  temperature_priority=High  temperature=300 K  temperature_nominal_specify=off  temperature_nominal_unit=K  temperature_nominal_value=1
      settings: InternalSimscapePortConfiguration="{\"Bottom\":[],\"Left\":[{\"id\":\"C\",\"label\":\"C\",\"type\":\"foundation.mechanical.rotational.rotational\"}],\"Right\":[{\"id\":\"P\",\"label\":\"P\",\"type\":\"foundation.mechanical.rotational.rotational\"},{\"id\":\"S\",\"label\":\"S\",\"type\":\"foundation.mechanical.rotational.rotational\"}],\"Top\":[]}"
  Torque Sensor : fl_lib/Mechanical/Mechanical Sensors/Ideal Torque Sensor
  Torque to Pressure : Subsystem
  S2 : PMIOPort  Side=Right
  S1 : PMIOPort  Port=2  Side=Right
  D : PMIOPort  Port=3  Side=Left
  connections:
  Input Pinion Crown Gear/RConn1 -- Disk Friction Clutch 1/LConn2 -- Sun-Planet Bevel 1/LConn1 -- Sun-Planet Bevel 2/LConn1 -- Disk Friction Clutch 2/LConn2
  S2/RConn1 -- Disk Friction Clutch 2/RConn1 -- Sun-Planet Bevel 2/RConn2
  S1/RConn1 -- Disk Friction Clutch 1/RConn1 -- Sun-Planet Bevel 1/RConn2
  Torque Sensor/RConn1 -- Input Pinion Crown Gear/LConn1
  D/RConn1 -- Torque Sensor/LConn1
  Sun-Planet Bevel 2/RConn1 -- Spring- Damper/RConn1
  Spring- Damper/LConn1 -- Sun-Planet Bevel 1/RConn1
  Disk Friction Clutch 1/LConn1 -- Torque to Pressure/RConn1 -- Disk Friction Clutch 2/LConn1
  Torque to Pressure/LConn1 -- Torque Sensor/RConn2

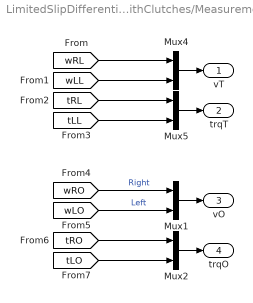
== system LimitedSlipDifferentialWithClutches/Measurements ==
  Mux{1..2,4..5} (4 alike) : Mux  Inputs=2
  vT : Outport  VectorParamsAs1DForOutWhenUnconnected=off
  trqT : Outport  Port=2  VectorParamsAs1DForOutWhenUnconnected=off
  vO : Outport  Port=3  VectorParamsAs1DForOutWhenUnconnected=off
  trqO : Outport  Port=4  VectorParamsAs1DForOutWhenUnconnected=off
  wires:
  Mux5/1 -> trqT/1
  Mux4/1 -> vT/1
  [wRL] -> Mux4/1
  [wLL] -> Mux4/2
  [tRL] -> Mux5/1
  [tLL] -> Mux5/2
  [wRO] -> Mux1/1  "Right"
  [wLO] -> Mux1/2  "Left"
  [tRO] -> Mux2/1
  [tLO] -> Mux2/2
  Mux1/1 -> vO/1
  Mux2/1 -> trqO/1
